simulink model "initial_PI_fzc"  (R2015a)
settings: Solver=ode45  StartTime=0.0  StopTime=10  RelTol=1e-3
libraries: fuzblock x1
settings Model: Creator=Home  LastModifiedBy=Home

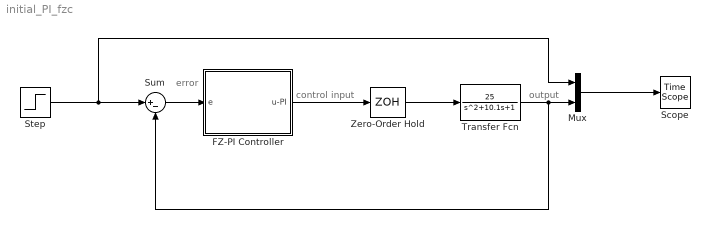
== system initial_PI_fzc ==
  note: output
  note: control input
  note: error
  FZ-PI Controller : Subsystem
  Mux : Mux  Inputs=2
  Scope : TimeScope
  Step : Step  Time=0  After=50  SampleTime=0
  Sum : Sum  Inputs=|+-
  Transfer Fcn : TransferFcn  Numerator=[25]  Denominator=[1 10.1 1]
  Zero-Order Hold : ZeroOrderHold  SampleTime=0.01
  wires:
  Mux/1 -> Scope/1
  Transfer Fcn/1 -> Sum/2, Mux/2
  Zero-Order Hold/1 -> Transfer Fcn/1
  Sum/1 -> FZ-PI Controller/1(e)
  Step/1 -> Mux/1, Sum/1
  FZ-PI Controller/1(u-PI) -> Zero-Order Hold/1

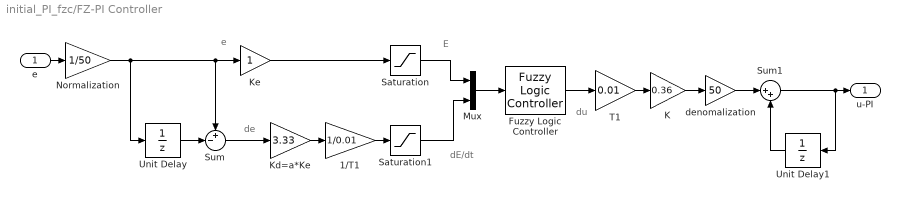
== system initial_PI_fzc/FZ-PI Controller ==
  note: du
  note: dE/dt
  note: E
  note: de
  note: e
  e : Inport
  1/T1 : Gain  Gain=1/0.01  OutDataTypeStr=Inherit: Same as input  ParamDataTypeStr=Inherit: Same as input
  Fuzzy Logic Controller : fuzblock/Fuzzy Logic  Controller  fis='fpi.fis'
  K : Gain  Gain=0.36  OutDataTypeStr=Inherit: Same as input  ParamDataTypeStr=Inherit: Same as input
  Kd=a*Ke : Gain  Gain=3.33  OutDataTypeStr=Inherit: Same as input  ParamDataTypeStr=Inherit: Same as input
  Ke : Gain  OutDataTypeStr=Inherit: Same as input  ParamDataTypeStr=Inherit: Same as input
  Mux : Mux  Inputs=2
  Normalization : Gain  Gain=1/50  OutDataTypeStr=Inherit: Same as input  ParamDataTypeStr=Inherit: Same as input
  Saturation : Saturate  UpperLimit=1  LowerLimit=-1
  Saturation1 : Saturate  UpperLimit=1  LowerLimit=-1
  Sum : Sum  Inputs=+-|
  Sum1 : Sum  Inputs=|++
  T1 : Gain  Gain=0.01  OutDataTypeStr=Inherit: Same as input  ParamDataTypeStr=Inherit: Same as input
  Unit Delay : UnitDelay  SampleTime=0.01
  Unit Delay1 : UnitDelay  SampleTime=0.01
  denomalization : Gain  Gain=50  OutDataTypeStr=Inherit: Same as input  ParamDataTypeStr=Inherit: Same as input
  u-PI : Outport
  wires:
  e/1 -> Normalization/1
  Normalization/1 -> Unit Delay/1, Sum/1, Ke/1
  Unit Delay/1 -> Sum/2
  Sum/1 -> Kd=a*Ke/1
  Kd=a*Ke/1 -> 1/T1/1
  1/T1/1 -> Saturation1/1
  Ke/1 -> Saturation/1
  Saturation/1 -> Mux/1
  Saturation1/1 -> Mux/2
  Mux/1 -> Fuzzy Logic Controller/1
  Fuzzy Logic Controller/1 -> T1/1
  T1/1 -> K/1
  K/1 -> denomalization/1
  denomalization/1 -> Sum1/1
  Sum1/1 -> u-PI/1, Unit Delay1/1
  Unit Delay1/1 -> Sum1/2
